simulink model "twelvepulses"  (Simulink 6.1)
settings: Solver=ode23tb  StartTime=0.0  StopTime=.1  RelTol=1e-3
undefined symbols (not defined in the file): D1, Delta
libraries: powerlib x16, powerlib_extras x1
settings Model: Creator=dkennedy  LastModifiedBy=ThinkPad  ExtModeAutoUpdateStatusClock=off
settings DataIOCC: SignalLoggingName=sigsOut
settings OptimizationCC: BlockReduction=off  BooleanDataType=off
settings HardwareCC: TargetUnknown=on

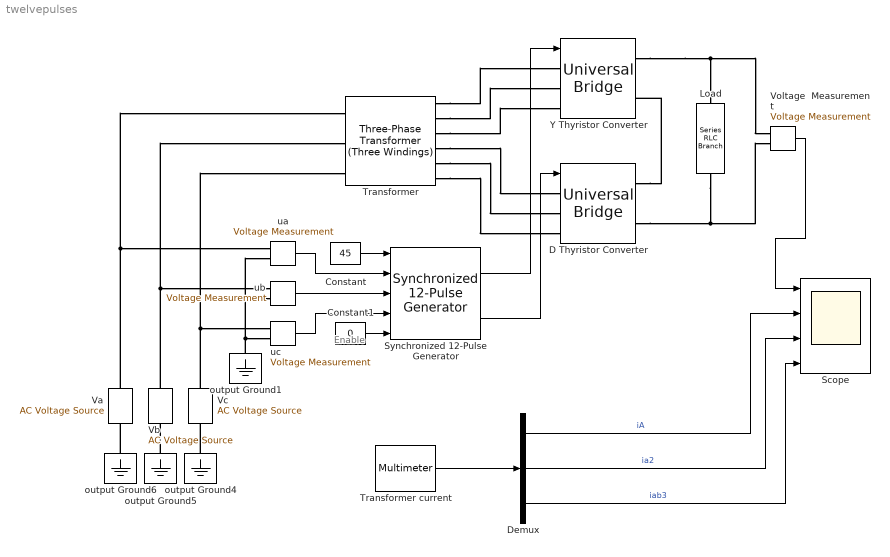
== system twelvepulses ==
  note: Enable
  " Synchronized 12-Pulse Generator" : powerlib_extras/Control  Blocks/ Synchronized 12-Pulse Generator  freq=50  pwidth=20  Double_Pulse=off
  Constant : Constant  Value=45
  Constant1 : Constant  Value=0
  D Thyristor Converter : powerlib/Power Electronics/Universal Bridge  Arms=3  SnubberResistance=2000  SnubberCapacitance=inf  Device=Thyristors  Ron=1e-3  Lon=0  ForwardVoltages="[  0.8  0.8  ]"  ForwardVoltage=0  GTOparameters=[ 10e-6 , 20e-6 ]  IGBTparameters=[ 1e-6 , 2e-6 ]  Measurements=None
  Demux : Demux  Outputs=3
  Load : powerlib/Elements/Series RLC Branch  Orientation=down  PhysicalDomain=powersysdomain  SubClassName=unknown  LeftPortType=p1  RightPortType=p1  LConnTagsString=__new0  RConnTagsString=__new0  Resistance=10  Inductance=0.1  Capacitance=inf  Measurements=None
  Scope : Scope  NumInputPorts=4
      settings: TimeRange=0.05  YMin=-400~-60~-60~-60  YMax=400~60~60~60  Decimation=5  SampleInput=on  SampleTime=1e-4
  Transformer : powerlib/Elements/Three-Phase Transformer (Three Windings)  NominalPower=[ 1200e6 , 50 ]  Winding1Connection=Yg  Winding1="[ 200e3 0  0 ]"  Winding2Connection=Y  Winding2=[ 200e3 0 0]  Winding3Connection=Delta (D1)  Winding3=[ 200e3 0.001 0]  SetSaturation=off  Rm=500  Lm=500  Saturation=[0 0; 1 1.2; 2 1.1]  Hysteresis=off  DataFile='basic_model'  SetInitialFlux=off  InitialFluxes=[0.8 -0.8 0.7]  Measurements=Winding currents  TransfoNumber=0
      settings: AttributesFormatString=\n
  "Transformer current " : powerlib/Measurements/Multimeter  Tag=PoWeRsYsTeMmEaSuReMeNt  PhasorSimulation=off  OutputType=Magnitude  sel=[1 4 7]  L=9  Gain=[1 -1 -1]  yselected={'Iag_w1: Transformer','Ian_w2: Transformer','Iab_w3: Transformer'};  PSBOutputType=1  PSBequivalent=0  AxesSetting=[0,0.1,-100,100]  Display=0  SavedBlockNames=-11
      settings: AttributesFormatString=\n
  Va : powerlib/Electrical Sources/AC Voltage Source  Description=source block  Orientation=up  Amplitude=100  Phase=0  Frequency=50  SampleTime=0  Measurements=None
      settings: AttributesFormatString=\n
  Vb : powerlib/Electrical Sources/AC Voltage Source  Description=source block  Orientation=up  Amplitude=100  Phase=-120  Frequency=50  SampleTime=0  Measurements=None
      settings: AttributesFormatString=\n
  Vc : powerlib/Electrical Sources/AC Voltage Source  Description=source block  Orientation=up  Amplitude=100  Phase=120  Frequency=50  SampleTime=0  Measurements=None
      settings: AttributesFormatString=\n
  Voltage  Measurement : powerlib/Measurements/Voltage Measurement  PhasorSimulation=off  OutputType=Complex  PSBequivalent=0
  Y Thyristor Converter : powerlib/Power Electronics/Universal Bridge  Arms=3  SnubberResistance=2000  SnubberCapacitance=.1e-6  Device=Thyristors  Ron=1e-3  Lon=0  ForwardVoltages="[  0.8  0.8  ]"  ForwardVoltage=0  GTOparameters=[ 10e-6 , 20e-6 ]  IGBTparameters=[ 1e-6 , 2e-6 ]  Measurements=None
  output Ground{1,4..6} (4 alike) : powerlib/Elements/Ground  Orientation=down  PhysicalDomain=powersysdomain  SubClassName=unknown  LeftPortType=p1  RightPortType=p1  LConnTagsString=a
  ua : powerlib/Measurements/Voltage Measurement  Tag=PoWeRsYsTeMmEaSuReMeNt  PhasorSimulation=off  OutputType=Magnitude  PSBequivalent=0
  ub : powerlib/Measurements/Voltage Measurement  Tag=PoWeRsYsTeMmEaSuReMeNt  PhasorSimulation=off  OutputType=Magnitude  PSBequivalent=0
  uc : powerlib/Measurements/Voltage Measurement  Tag=PoWeRsYsTeMmEaSuReMeNt  PhasorSimulation=off  OutputType=Magnitude  PSBequivalent=0
  wires:
  Constant1/1 -> " Synchronized 12-Pulse Generator"/5
  Constant/1 -> " Synchronized 12-Pulse Generator"/1
  ua/1 -> " Synchronized 12-Pulse Generator"/2
  ub/1 -> " Synchronized 12-Pulse Generator"/3
  uc/1 -> " Synchronized 12-Pulse Generator"/4
  " Synchronized 12-Pulse Generator"/1 -> Y Thyristor Converter/1
  " Synchronized 12-Pulse Generator"/2 -> D Thyristor Converter/1
  Demux/1 -> Scope/2  "iA"
  Demux/2 -> Scope/3  "ia2"
  "Transformer current "/1 -> Demux/1
  Voltage  Measurement/1 -> Scope/1
  Demux/3 -> Scope/4  "iab3"
  connections:
  Vc/RConn1 -- uc/LConn1 -- Transformer/LConn3
  Vb/RConn1 -- ub/LConn1 -- Transformer/LConn2
  Va/RConn1 -- ua/LConn1 -- Transformer/LConn1
  output Ground1/LConn1 -- ua/LConn2 -- ub/LConn2 -- uc/LConn2
  D Thyristor Converter/RConn1 -- Y Thyristor Converter/RConn2
  D Thyristor Converter/RConn2 -- Voltage  Measurement/LConn2 -- Load/RConn1
  Transformer/RConn2 -- Y Thyristor Converter/LConn2
  Transformer/RConn1 -- Y Thyristor Converter/LConn1
  Transformer/RConn3 -- Y Thyristor Converter/LConn3
  Y Thyristor Converter/RConn1 -- Load/LConn1 -- Voltage  Measurement/LConn1
  Transformer/RConn4 -- D Thyristor Converter/LConn1
  Transformer/RConn5 -- D Thyristor Converter/LConn2
  Transformer/RConn6 -- D Thyristor Converter/LConn3
  output Ground4/LConn1 -- Vc/LConn1
  output Ground5/LConn1 -- Vb/LConn1
  output Ground6/LConn1 -- Va/LConn1
